simulink model "magNoise"  (R2013a)
settings: Solver=ode45  StartTime=0.0  StopTime=t  RelTol=1e-3
values from neighbouring files (symbols this model uses):
  sampleTime = 0.01    [workspace.mat]
libraries: simulink x4
settings Model: Creator=User  LastModifiedBy=User

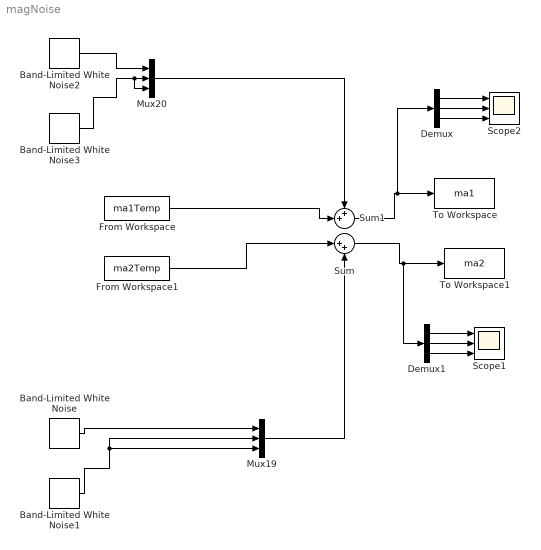
== system magNoise ==
  Band-Limited White Noise : simulink/Sources/Band-Limited White Noise  Cov=[0.01*0.8671E-5*0.5]  Ts=sampleTime  seed=[23341]
  Band-Limited White Noise1 : simulink/Sources/Band-Limited White Noise  Cov=[0.01*0.8671E-5*0.5]  Ts=sampleTime  seed=[23341]
  Band-Limited White Noise2 : simulink/Sources/Band-Limited White Noise  Cov=[0.01*0.0561E-4*0.5]  Ts=sampleTime  seed=[23341]
  Band-Limited White Noise3 : simulink/Sources/Band-Limited White Noise  Cov=[0.01*0.0724E-4*0.5]  Ts=sampleTime  seed=[23341]
  Demux : Demux  Outputs=3
  Demux1 : Demux  Outputs=3
  From Workspace : FromWorkspace  VariableName=ma1Temp  SampleTime=sampleTime
  From Workspace1 : FromWorkspace  VariableName=ma2Temp  SampleTime=sampleTime
  Mux19 : Mux  Inputs=3
  Mux20 : Mux  Inputs=3
  Scope1 : Scope  NumInputPorts=3
      settings: YMin=-5~-5~-5  YMax=5~5~5
  Scope2 : Scope  NumInputPorts=3
      settings: YMin=-5~-5~-5  YMax=5~5~5
  Sum : Sum  Inputs=|++
  Sum1 : Sum  Inputs=++|
  To Workspace : ToWorkspace  VariableName=ma1  SampleTime=sampleTime  SaveFormat=Structure With Time
  To Workspace1 : ToWorkspace  VariableName=ma2  SampleTime=sampleTime  SaveFormat=Structure With Time
  wires:
  Band-Limited White Noise/1 -> Mux19/1
  Band-Limited White Noise1/1 -> Mux19/3, Mux19/2
  Band-Limited White Noise2/1 -> Mux20/1
  Band-Limited White Noise3/1 -> Mux20/3, Mux20/2
  Mux20/1 -> Sum1/1
  Mux19/1 -> Sum/2
  From Workspace/1 -> Sum1/2
  From Workspace1/1 -> Sum/1
  Sum1/1 -> Demux/1, To Workspace/1
  Sum/1 -> Demux1/1, To Workspace1/1
  Demux1/1 -> Scope1/1
  Demux1/2 -> Scope1/2
  Demux1/3 -> Scope1/3
  Demux/1 -> Scope2/1
  Demux/2 -> Scope2/2
  Demux/3 -> Scope2/3
